simulink model "Bait_Ambrosino_hinf"  (R2025b)
settings: Solver=VariableStepAuto  StartTime=0.0  StopTime=10.0  RelTol=1e-3
undefined symbols (not defined in the file): A, B, C, nu, ny, xref
libraries: cstblocks x2
settings Model: Creator=Miche  LastModifiedBy=Miche

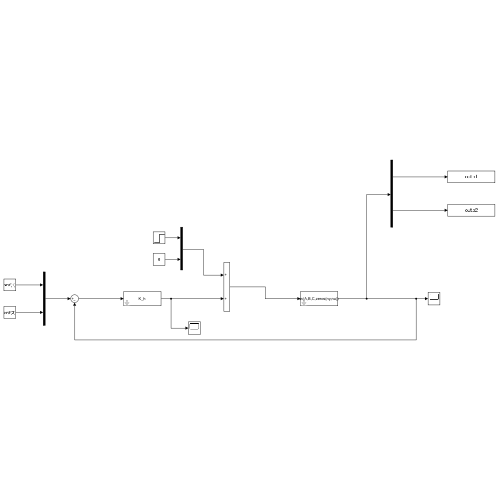
[thumbnail: Simulink's stored preview of the top-level diagram]
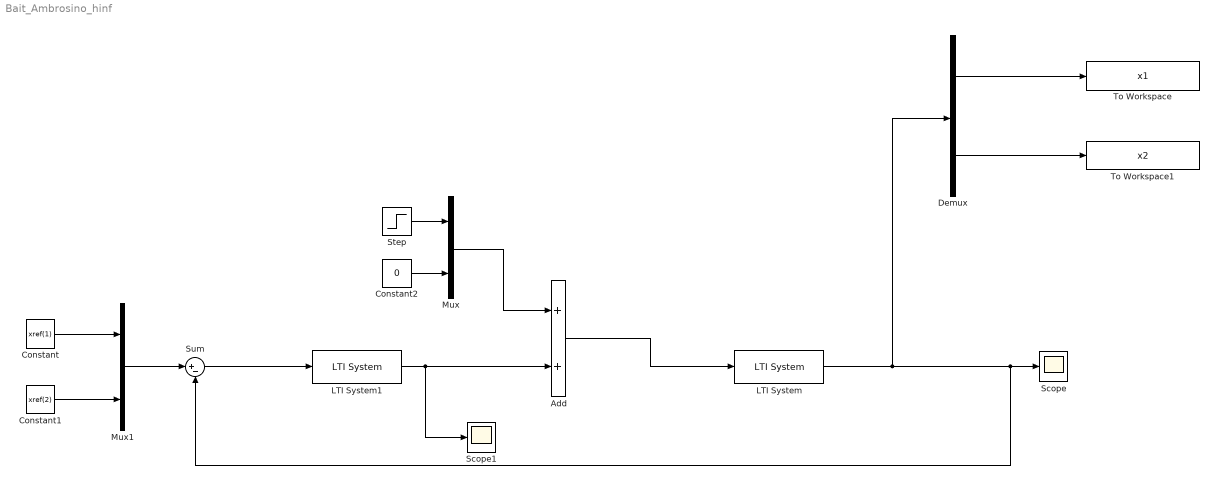
== system Bait_Ambrosino_hinf ==
  Add : Sum
  Constant : Constant  Value=xref(1)
  Constant1 : Constant  Value=xref(2)
  Constant2 : Constant  Value=0
  Demux : Demux  Outputs=2
  LTI System : cstblocks/LTI System  sys=ss(A,B,C,zeros(ny,nu))  IC=[]  PadeOrder=0
  LTI System1 : cstblocks/LTI System  sys=K_h  IC=[]  PadeOrder=0
  Mux : Mux  Inputs=2
  Mux1 : Mux  Inputs=2
  Scope : Scope
      settings: ActiveDisplayYMinimum=-0.16521840755390069  ActiveDisplayYMaximum=1.066702724717902
  Scope1 : Scope
      settings: ActiveDisplayYMinimum=-9.0728220080868169  ActiveDisplayYMaximum=34.867561279040807
  Step : Step  After=0.75  SampleTime=0
  Sum : Sum  Inputs=|+-
  To Workspace : ToWorkspace  VariableName=x1  SaveFormat=Timeseries  SampleTime=-1
  To Workspace1 : ToWorkspace  VariableName=x2  SaveFormat=Timeseries  SampleTime=-1
  wires:
  Sum/1 -> LTI System1/1
  Mux1/1 -> Sum/1
  Constant/1 -> Mux1/1
  Constant1/1 -> Mux1/2
  Constant2/1 -> Mux/2
  Step/1 -> Mux/1
  LTI System1/1 -> Scope1/1, Add/2
  Mux/1 -> Add/1
  Add/1 -> LTI System/1
  Demux/2 -> To Workspace1/1
  LTI System/1 -> Demux/1, Scope/1, Sum/2
  Demux/1 -> To Workspace/1
